simulink library "marine_gnc"  (Simulink 7.4)
settings: Solver=ode45  SolverMode=SingleTasking  StartTime=0.0  StopTime=10.0  RelTol=1e-3
undefined symbols (not defined in the file or in its folder): CN_data, CX_data, CY_data, D, G, K_supply, kt2ms, M, MA, magnitude, marine, Models, MRB, order, pathlength, RAO_Amp, RAO_Dir, RAO_Freq, RAO_Phase, RAO_Vel, RAO_yaw_back, RAO_yaw_quant, RAO_yaw_quantization_flag, rho_a, Semi, sub, T_supply, table, Tanker, vessel, Vessels
libraries: marine_gnc x64, simulink x39, cybersealib x1
(part 1 of 6)
settings Model: Creator=tristan  LastModifiedBy=Thor

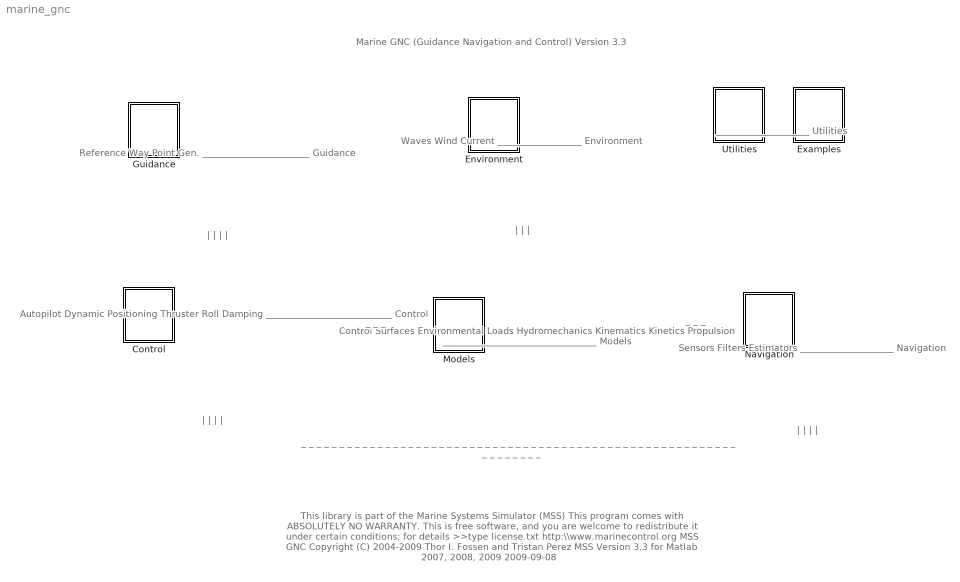
== system marine_gnc ==
  note: Marine GNC (Guidance Navigation and Control) Version 3.3
  note: Reference
      |                      Way Point Gen.
      |
      |
      | _______________________
      | Guidance
  note: Control Surfaces
      |                              Environmental Loads
      |                      Hydromechanics
      |           Kinematics
      |      Kinetics
      |            Propulsion
      | _________________________________
      | Models
  note: Autopilot
      |                          Dynamic Positioning
      |     Thruster
      |              Roll Damping
      | ___________________________
      | Control
  note: Waves
      |                    Wind
      |                        Current
      |
      | __________________
      | Environment
  note: |
      | |
      | |
  note: _ _ _
  note: _ _ _
  note: |
      | |
      | |
      | |
  note: |
      | |
      | |
      | |
  note: |
      | |
      | |
      | |
  note: _ _ _ _ _ _ _ _ _ _ _ _ _ _ _ _ _ _ _ _ _ _ _ _ _ _ _ _ _ _ _ _ _ _ _ _ _ _ _ _ _ _ _ _ _ _ _ _ _ _ _ _ _ _ _ _ _ _ _ _ _ _ _ _ _
  note: Sensors
      |                    Filters
      |                           Estimators
      |
      | ____________________
      | Navigation
  note: This library is part of the Marine Systems Simulator (MSS)
      | This program comes with ABSOLUTELY NO WARRANTY. This is free software,
      | and you are welcome to redistribute it under certain conditions; for details
      | >>type license.txt
      |
      |  http:\\www.marinecontrol.org
      |
      | MSS GNC  Copyright (C) 2004-2009 Thor I. Fossen and Tristan Perez
      |  MSS Version 3.3 for Matlab 2007, 2008, 2009
      | 2009-09-08
  note: ____________________
      | Utilities
  Control : Subsystem
  Environment : Subsystem
  Examples : Subsystem  AncestorBlock=Marine_GNC/Support and Examples
  Guidance : Subsystem
  Models : Subsystem
  Navigation : Subsystem
  Utilities : Subsystem

== system marine_gnc/Control ==
  Autopilots : Subsystem
  "Dynamic  Positioning " : Subsystem
  Thruster : Subsystem

== system marine_gnc/Environment ==
  Current : Subsystem
  Waves : Subsystem
  Wind : Subsystem

== system marine_gnc/Examples ==
  Applications : Subsystem
  Vessels : Subsystem

== system marine_gnc/Guidance ==
  Reference model : Subsystem  mask(3rd-order reference model){v_max=1.0, zeta_d=1.0, w_d=0.1}
      mask prompts: v_max "Max. velocity:"; zeta_d "Relative damping ratio:"; w_d "Natural frequency:"
      mask help: 3rd-order reference model with velocity saturation.
      mask Display:
      | disp('3rd order \nLP-filter')
      | port_label('output', 3, 'acc_d')
      | port_label('output', 2, 'vel_d')
      | port_label('output', 1, 'mag_d')
      | port_label('input', 1, 'ref')
  Way-point guidance block : Subsystem  mask(Guidance){x_vector=[-800 -500 -200 -50 -200 -250 200 500 500 300 0 -300 -600], y_vector=[100 1800 2000 1500 1000 100 1000 300 -250 -200 100 -600 -1000], method=5th order polynomial, drawmode=off, stop=on, mode=Acc, start=[100 0], final=[0 100], constraint=off}
      mask prompts: x_vector "X value"; y_vector "Y value"; method "Computation method for path generation"; drawmode "Draw an extra plot showing the path with waypoints"; stop "Stop simulation when last waypoint is reached"; mode "Use constraints on acceleration or velocity in the endpoints"; start "Constraints in first waypoint [x, y]. (Only applicable for cubic splines)"; final "Constraints in last waypoint [x, y]. (Only applicable for cubic splines)"; constraint "Use constraints on the derivatives (Only applicable for 5th order)"
      mask help:
      | Way-Point Guidance Block
      | Author:  Jorgen Corneliussen
      | Date:     20 November 2002
      |
      | Creates a three times differentiable path between the waypoints provided. The user can choose between cubic splines and polinomial interpolation.
      |
      | NOTE: You have to supply the actual waypoints for the path generation.
      mask init:
      | if method == 1
      | 	[table, pathlength] = order3(x_vector,y_vector, drawmode, mode, start(1), final(1), start(2), final(2));
      | elseif method == 2
      | 	[table, pathlength] = order5(drawmode, constraint, x_vector, y_vector);
      | else
      | 	disp('Error in block initialization')
      | end
      mask Help:
      | <p>Way-Point Guidance Block<br>
      |   Author: Jorgen Corneliussen<br>
      |   Date: 20 November 2002</p>
      | <ul>
      |   <li> The input vectors must be of the same length, and contain the coordinates
      |     of the waypoints.</li>
      |   <li>If chosen, the block can draw an extra plot showing the path and the waypoints.</li>
      |   <li> The field &quot;Computation method&quot; allows the user to choose between
      |     a third and fifth order polynomal for path generation. </li>
      |   <li>If &quot;Stop simulation&quot; is not checked, the velocity input to the
      |     block is set to zero when the last waypoint is reached. </li>
      |   <li>For the third order algorithm, the user can choose between having endpoint
      |     constraints in velocity or acceleration. The values must be provided in the
      |     specified fields.</li>
      |   <li>For the fifth order polynomial, the user can choose to constrain the derivatives
      |     in the waypoints. This might in some cases reduce oscillations.<br>
      |   </li>
      | </ul>
      mask StyleString: edit,edit,popup(Cubic spline|5th order polynomial),checkbox,checkbox,popup(Vel|Acc),edit,edit,checkbox
      mask Display:
      | image(imread('compass.jpg'))
      | 
      | color('black'); port_label('output', 1, 'xy')
      | color('black'); port_label('output', 2, 'eta_vec')
      | color('black'); port_label('output', 3, 'vs_tot')
      | 
      | color('black'); port_label('input', 1, 'ud_total')
      | color('black'); port_label('input', 2, 'theta')
  "Zig-Zag test rudder command " : Subsystem  mask(Z- Manoeuvre test or Zig-Zag test){RL=}
      mask prompts: RL "Maximum rudder angle [rad]:"
      mask help:
      | This block generates the rudder command for a Z-manoeuvre test
      | IMO A601, ITTC 1975, SNAME 1989.
      | Copyright (C) 2005 NTNU
      |  Author: Tristan Perez

== system marine_gnc/Models ==
  " Kinematics" : Subsystem
  " Kinetics " : Subsystem
  Control Surfaces : Subsystem
  Environmental Loads : Subsystem
  Hydromecanics : Subsystem
  Propulsion : Subsystem

== system marine_gnc/Navigation ==
  Filters : Subsystem
  Observers : Subsystem
  "Sensors " : Subsystem

== system marine_gnc/Utilities ==
  Dynamics : Subsystem
  Math Operations : Subsystem
  Simulation tools : Subsystem
  Visualization : Subsystem

== system marine_gnc/Control/Autopilots ==
  Heading autopilot : Subsystem  mask(Course Autopilot){T_nomoto=1, K_nomoto=1, Kp=1, Td=0, Ti=0}
      mask prompts: T_nomoto "Nomoto Time Constant: T"; K_nomoto "Nomoto gain: K"; Kp "Proportional Gain: Kp"; Td "Derivative Time: Td"; Ti "Integral Time: Ti"
      mask help: PID Autopilot with reference feedforward.
      mask Help: INPUTS: (1)  desired position, (2) desired velocity, (3) desired acceleration, (4) heading angle, (5) heading rate: OUTPUTS: (1) rudder angle
      mask Display: disp('PID\n tracking\n controller')

== system marine_gnc/Control/Dynamic  Positioning  ==
  DP controller : Subsystem  mask(Nonlinear DP Controller){Kp=diag([1 1 1]), Kd=diag([1 1 1]), Ki=diag([1 1 1])}
      mask prompts: Kp "Proportional Gain Matrix: Kp"; Kd "Derivative Gain Matrix: Kd"; Ki "Integral Gain Matrix: Ki"
      mask help: Nonlinear PID controller for Set-Point Reulation in Surge, Sway and Yaw
      mask Help:
      | The nonlinear  PID controller uses the rotation matrix in yaw for proper scaling of the surge, sway and yaw gains as a function of the yaw angle.
      | INPUTS: (1) eta_ref, (2) eta, (3) nu. OUPUTS: (1) tau.
      mask Display: disp('Nonlinear PID\n set-point controller')

== system marine_gnc/Control/Thruster ==

== system marine_gnc/Environment/Current ==
  North-East current : Subsystem

== system marine_gnc/Environment/Waves ==
  " Gaussian Random Process" : Subsystem  AncestorBlock=|  mask(Gaussian Random Process as a Sum of Sinusoids){areg=, freq=, phases=}
      | dcmv/Environmental
      | Disturbances/Fourier representation of 
      | a Gaussian Random Process
      mask prompts: areg "Vector of Amplitudes [A1;A2;...]:"; freq "Vector of frequencies [W1;W2;...]  [rad/sec]:"; phases "Vector of random phases [P1;P2;...]  [rad]:"
      mask help:
      | y = Sum_i  Ai *cos(w_i*t+ Phi_i)
      | Input:
      |  t --Simulation time from a clock block
      | Output:
      |  y--Realization of the random process y(t) (time series)
      | Dependency: None
      |
      | Copyright (C), NTNU  2004
      | Author: Tristan Perez
      mask Help: web(['file:///' which('Help_Gaussian_Random_Process.htm')]);
      mask Display:
      | plot([-ones(1,17)
      | 	0.6333
      |      -1.5315
      |    -0.5146
      |     0.5573
      |     1.2590
      |     1.8899
      |     1.5451
      |    -0.1055
      |    -1.0617
      |    -1.3645
      |    -1.3826
      |    -1.2742
      |     0.3850
      |     1.0225
      |     1.1108
      |     1.1270
      |     0.3762
      |    -0.6570
      |    -1.1216
      |    -0.2885
      |     0.9176
      |     0.7826
      |    -0.3229
      |    -1.2406
      |    -0.9331
      |    -0.2407
      |     0.4134
      |     0.8612
      |     0.3025
      |     0.2761
      |     0.3856
      |     0.3689
      |    -0.0188
      |     0.3654
      |    -0.4219
      |    -1.0260
      |    -1.3896
      |    -0.6530
      |     0.2512
      |     1.0351
      |     1.6496
      |     0.8313
      |    -1.2176
      |    -1.0937
      |     0.0268
      |     1.0361
      |     1.1728
      |    -0.2176
      |    -0.6390
      |    -1.1209
      |    -1.0516
      |    -0.4193
      |     0.7858
      |     0.8509
      |     0.4288
      |     0.0431
      |     0.0587 -ones(1,15
      | 	)])
      | port_label('input',1,'time')
      | port_label('output',1,'y')
  Encounter frequency correction : Subsystem
      mask Type: Encounter frequency correction
      mask Description:
      | This block transforms the frequencies and wave numbers in the Waves bus generated by the MSS Waves block to encounter frequencies and encounter wave numbers using the transformation:
      | 
      | Omega_e = Omega - U*Omega^2*cos(Psi_r)/g
      | 
      | where U is the vessel forward speed, Psi_r is the angle of the waves relative to the vessel.
      | 
      | Inputs:
      | Waves - Bus of harmonic wave components generated by the MSS Waves block.
      | U          - Forward speed of the reference frame relative to NED (m/s) (Usually the low-frequency speed of the vessel)
      | Psi       - Yaw orientation of the reference frame relative to NED (rad) (Usually the low-frequency heading of the vessel)
      | 
      | Outputs:
      | Waves - Bus of harmonic wave components with corrected wave frequencies and wave numbers.
      | 
      | Copyright (C) 2005, NTNU
      | Author: Øyvind Notland Smogeli
  Linear 2nd-order  wave spectrum : Subsystem  mask{sigma=1, w_0=1, lambda=0.1}
      mask prompts: sigma "Wave spectrum gain: sigma  (m)"; w_0 "Wave spectrum peak frequency: w_0  (rad/s)"; lambda "Rrelative damping ratio: lambda"
      mask init:
      | w = 0.01:0.1:3*w_0;
      mask Display:
      | plot(w,4*w_0*sigma^2.*w.^2./((w_0^2-w.^2).^2+4*(lambda*w_0.*w).^2))
      | port_label('input', 1, 'w')
      | port_label('output', 1, 'y')
  W_wave 2 W_enc (no absolute value) : Subsystem
      mask Type: Wave frequency to Encounter Frequency
      mask Description:
      | This block implements the transformation:
      | 
      | We = W -U W^2 cos(Enc Aang) /g
      | 
      | Inputs:
      | U---forward speed of the reference frame (m/sec) (sually the speed of the vessel)
      | W--vector of wave frequencies (rad/sec)
      | Enc. Angle-- (rad) convention: 0-following seas; pi/2-port beam seas; pi-head seas
      | 
      | Outputs:
      | We--vector of encounter frequencies (rad/sec).
      | Ke-- vector of encounter wave numbers (Ke = We^2/g deep water assumption)
      | Copyright (C) 2005, NTNU
      | Author: Tristan Perez
      mask Help:
      | <p>This block implements the transformation: <br>
      | <br>
      | We = W -U W^2 cos(Enc Ang) /g <br>
      | <br>
      | Inputs:<br>
      | U---forward speed of the reference frame (m/sec) (Usually the speed of the
      | vessel)<br>
      | W--vector of wave frequencies (rad/sec)<br>
      | Enc. Angle-- (rad) convention: 0-following seas; pi/2-port beam seas; pi-head
      | seas<br>
      | <br>
      | Outputs:<br>
      | We--vector of encounter frequencies (rad/sec).<br>
      | Ke-- vector of encounter wave numbers (Ke = We^2/g deep water assumption)<br>
      | Copyright (C) 2005, NTNU<br>
      | Author: Tristan Perez </p>
  Wave velocitycalc : Subsystem
      mask Type: Wave velocitycalc
      mask Description: Caclulates the wave-induced water velocity in NED coordinates and surface elevation Zeta at the point [x y z] in NED. The Waves bus generated by the Waves module is needed as input.
  Waves : Subsystem  mask(Waves){spectrum_type=ITTC, disp_flag=on, plot_spectrum=off, plot_realization=off, hs=0.8, omega_peak=0, psi_mean=0, gamma=-1, spread=2, depth=inf, nfreq=20, ndir=10, energylim=0.005, freq_cutoff=3, dir_cutoff=0, rand_seed=123, rand_freq=on, rand_dir=on, Zeta_a=0, Omega=0, Phase=0, Wavenum=0, Psi=0}
      mask prompts: spectrum_type "Spectrum type"; disp_flag "Display initialization info in workspace window"; plot_spectrum "Plot spectrum"; plot_realization "Plot sea state realization (time-consuming)"; hs "Significant wave height Hs (m)"; omega_peak "Peak frequency omega_0 (rad/s)"; psi_mean "Mean wave direction (rad)"; gamma "Spectrum peakedness factor [1,7], 3.3 default, 0 for using DNV value"; spread "Wave spreading factor (1,2,3,4,5)"; depth "Average water depth (m), use inf for deep water"; nfreq "Number of frequencies in grid (recommended > 20)"; ndir "Number of directions in grid, 1 for long-crested waves"; energylim "Wave component energy limit [0 1] or number of waves (e.g. 50)"; freq_cutoff "Frequency cutoff factor [1.5, 5], default 3"; dir_cutoff "Direction cutoff [0, 3pi/8], default 0"; rand_seed "Random seed"; rand_freq "Random frequencies"; rand_dir "Random directions"; Zeta_a "Amplitude vector 'Zeta_a' (m)"; Omega "Frequency vector 'Omega' (rad/s)"; Phase "Phase vector 'Phase' (rad)"; Wavenum "Wavenumber vector 'Wavenum' (1/m)"; Psi "Direction vector 'Psi'  (rad)"
      mask help:
      | Calculate harmonic wave component parameters from a wave spectrum.
      | - Input one wave direction in the mask to get long-crested waves.
      | - Input zero peak frequency to get an expectation value from north sea statistical data.
      | - Input an integer > 1 for energylim to set the number of wave components fixed to nwaves = energylim.
      |
      | Copyright (C) 2004 NTNU
      | Author: Oyvind Notland Smogeli
      mask init:
      | if spectrum_type < 4
      | 	[Zeta_a, Omega, Phase, Wavenum, Psi] = Wave_init(spectrum_type, hs, omega_peak, psi_mean,...
      | 	gamma, spread, depth, nfreq, ndir, energylim, freq_cutoff, dir_cutoff, rand_freq, rand_dir,...
      | 	rand_seed, plot_spectrum, plot_realization, disp_flag);
      | end
      mask Help:
      | <font face="Arial">
      | <b>Project:</b> Marine Systems Simulator: MSS<br>
      | <br>
      | Define harmonic wave components describing the sea state by extracting
      | components from a given frequency and direction spectrum. The output from the
      | block is a bus containing the following wave parameter vectors:</font></p>
      | <p><font face="Arial"><b>Zeta_a</b>: Vector of harmonic wave amplitudes [m]<br>
      | <b>Omega: </b>Vector of harmonic wave frequencies [rad/s]<br>
      | <b>Phase: </b>Vector of harmonic wave phases (random) [rad]<br>
      | <b>Wavenum:</b> Vector of harmonic wave numbers [1/m]<br>
      | <b>Psi: </b>Vector of harmonic wave directions [rad]</font></p>
      | <p><font face="Arial">The time series of sea surface elevation Zeta(x,y,t) can
      | be obtained as</font></p>
      | <p><font face="Arial">Zeta(x,y,t) = Sum( Zeta_a(i)*cos(Omega(i)*t + Phase(i) - Wavenum(i)*(x*cos(Psi(i))
      | + y*sin(Psi(i)))) )</font></p>
      | <p><font face="Arial">where the sum is taken from i = 1 to i = n and n is the number of harmonic
      | wave components.</font></p>
      | <p>&nbsp;</p>
      | <p><font face="Arial">Input one wave direction to get long-crested waves.<br>
      | <br>
      | If the peak frequency is set to zero, then the peak frequency is obtained from
      | the sugnificant wave height usign a formula for the North Sea (Norsok):</font></p>
      | <p><font face="Arial">w0 = 2*pi/(4.883 + 2.68*Hs^0.54);</font></p>
      | 
      | <p>&nbsp;</p>
      | <p><font face="Arial">The energy limit (energylim) should be defined either as a positive factor
      | between 0 and 1, or as a positive integer. In the first case it will
      | discard all wave components with energy content less than this ratio of the
      | total energy content of the sea state. A recommended value is 0.005 or lower. In
      | the second case it will keep the nwaves = energylim most significant waves.</font></p>
      | <p>&nbsp;</p>
      | <p><font face="Arial">The wave elevation Zeta(x,y,t) at time t and at the coordinate (x,y) is found from the output vectors as:</font></p>
      | <p>&nbsp;</p>
      | <p><font face="Arial" color="#800000">References</font><ul>
      |   <li><font face="Arial">Sørensen, A.J. (2005) Lecture notes of TMR4240 &quot;Marine Cybernetics - Modelling and Control&quot;</font>
      |   <font face="Arial">Dept of Marine Technology NTNU.</font></li>
      |   <li><font face="Arial">Johannessen, K., T. S. Meling, S. Haver. Joint
      |   Distribution for Wind and<br>
      |   Waves in the Northern North Sea. IJOPE Vol. 12, No. 1, March 2002</font></li>
      |   <li>&nbsp;</li>
      |   </ul>
      | <p><font face="Arial">Johannessen, K., T. S. Meling, S. Haver. Joint
      | Distribution for Wind and<br>
      | Waves in the Northern North Sea. IJOPE Vol. 12, No. 1, March 2002</font><p>&nbsp;<p>
      |   <font face="Arial"><b>Author:</b> Øyvind Smogeli, September 2004 </font>
      | <p>&nbsp;</p>
      | <p>&nbsp;</p>
      mask StyleString: popup(ITTC|Jonswap|Torsethaugen|Predefined waves),checkbox,checkbox,checkbox,edit,edit,edit,edit,edit,edit,edit,edit,edit,edit,edit,edit,checkbox,checkbox,edit,edit,edit,edit,edit
      mask CallbackString: Wave_callback;||||||||||||||||||||||

== system marine_gnc/Environment/Wind ==
  Wind : Subsystem  mask(Wind){page=1, Par_Wind_slowlyvar=off, Par_Wind_gust=off, Par_Wind_V=10, Par_Wind_angle=0, Par_Wind_spectrum_type=1, Par_Wind_z=10, Par_Wind_sample_time=0.1, Par_Wind_speed_T=10, Par_Wind_angle_T=10, Par_Wind_speed_noise_pow=1, Par_Wind_angle_noise_pow=0.01, Par_Wind_speed_rand_max=1, Par_Wind_angle_rand_max=pi/4, Par_Wind_speed_seed=123, Par_Wind_angle_seed=321, Par_Wind_phase_seed=1532, Par_Wind_kappa_H=0.0026, Par_Wind_L=1800, Par_Wind_minfreq=1E-4, Par_Wind_maxfreq=0.1, Par_Wind_nfreq=100}
      mask prompts: Par_Wind_slowlyvar "Include slowly-varing wind velocity and direction"; Par_Wind_gust "Include wind gust"; Par_Wind_V "Mean wind velocity [m/s]"; Par_Wind_angle "Mean wind angle [rad]"; Par_Wind_spectrum_type "Wind gust spectrum type"; Par_Wind_z "Height over water surface [m (for NORSOK wind spectrum)]"; Par_Wind_sample_time "Wind sample time [s]"; Par_Wind_speed_T "Wind speed time constant [s]"; Par_Wind_angle_T "Wind angle time constant [s]"; Par_Wind_speed_noise_pow "Wind speed noise power"; Par_Wind_angle_noise_pow "Wind angle noise power"; Par_Wind_speed_rand_max "Wind speed saturation [m/s] (max random variation about mean)"; Par_Wind_angle_rand_max "Wind angle saturation [rad] (max random variation about mean)"; Par_Wind_speed_seed "Wind speed random seed"; Par_Wind_angle_seed "Wind angle random seed"; Par_Wind_phase_seed "Wind gust phase seed"; Par_Wind_kappa_H "Sea surface drag coefficient for Harris wind spectrum (0.0026)"; Par_Wind_L "Scaling length for Harris wind spectrum (1800)"; Par_Wind_minfreq "Minimum frequency in gust [Hz] (1E-4)"; Par_Wind_maxfreq "Maximum frequency in gust [Hz] (0.1)"; Par_Wind_nfreq "Number of frequency components"
      mask help:
      | Generates wind speed and direction based on the mean angle and mean wind speed at 10 meters height. The total velocity is composed of a slowly-varying mean superposed with gusts based on a chosen wind spectrum. The direction is slowly-varying based on a random process.
      |
      | The wind spectrum types are:
      |
      | 1) Harris         (based on measurements over land)
      | 2) NORSOK   (based on measurements from the North Sea)
      mask Help:
      | <b>Part of the Marine Systems Simulator: MSS</b><p>Generate wind speed and direction based on the mean angle and mean wind
      | speed at 10 meters height. The total velocity is composed of a slowly-varying
      | mean superposed with gusts based on a chosen wind spectrum. The direction is
      | slowly-varying based on a random process.<br>
      | <br>
      | The wind spectrum types are:<br>
      | <br>
      | 1) Harris (based on measurements over land)<br>
      | 2) NORSOK (based on measurements from the North Sea)</p>
      | <p>The wind gust from the Harris spectrum is uniform over the height, whereas
      | the wind gust from the NORSOK spectrum varies with the height.</p>
      | <p>The random variation of the mean speed and angle can be limited by two saturation
      | parameters, which define the maximum random deviation from the mean value.<p><b>Outputs:
      | </b> </p>
      | <p>angle: [rad] Wind angle in the n-frame<br>
      | speed: [m/s] Wind velocity in the n-frame<p>
      | <b>Copyright NTNU 2005</b></p>
      | <p><b>Author:</b> Oyvind N. Smogeli, 2005-05-03</p>
      mask StyleString: popup(1|2),checkbox,checkbox,edit,edit,popup(1|2),edit,edit,edit,edit,edit,edit,edit,edit,edit,edit,edit,edit,edit,edit,edit,edit
      mask CallbackString: MSS_mask_page(12);|||||||||||||||||||||

== system marine_gnc/Examples/Applications ==
  Autopilot - Kalman filter based wave filter using only compass : Subsystem  AncestorBlock=marine/Examples/Autopilot - Kalman filter based wave filter using only compass  mask{A=}
      mask prompts: A "Needed to invoke OpenFcn from the browser:"
      settings: OpenFcn=sfundemo_open('demowf3')
      mask Display: disp('Autopilot - \n Kalman filter based\n wave filter using\n only compass');
  Autopilot - passive wave filter using compass/gyro : Subsystem  mask{A=}
      mask prompts: A "Needed to invoke OpenFcn from the browser:"
      settings: OpenFcn=sfundemo_open('demowf2')
      mask Display:
      | disp('Autopilot - \n passive wave filter\n
      | using compass/gyro');
  Autopilot - passive wave filter using only compass : Subsystem  mask{A=}
      mask prompts: A "Needed to invoke OpenFcn from the browser:"
      settings: OpenFcn=sfundemo_open('demowf1')
      mask Display:
      | disp('Autopilot - \n passive wave filter \n
      | using only compass');
  DP system for CyberShipII : Subsystem  mask{A=}
      mask prompts: A "Needed to invoke OpenFcn from the browser:"
      settings: OpenFcn=sfundemo_open('demoCS2')
      mask Display: disp('DP system for \n CyberShipII');
  DP system for semi-submersible : Subsystem  mask{A=}
      mask prompts: A "Needed to invoke OpenFcn from the browser:"
      settings: OpenFcn=sfundemo_open('demorig')
      mask Display: disp('DP system for\n semi-submersible');
  Simulink interface for m-file vessel models : Subsystem  mask{A=}
      mask prompts: A "Needed to invoke OpenFcn from the browser:"
      settings: OpenFcn=sfundemo_open('demomf')
      mask Display:
      | disp('Simulink interface for\n
      | m-file vessel models');
  Thruster configuration demo for a supply vessel : Subsystem  mask{A=}
      mask prompts: A "Needed to invoke OpenFcn from the browser:"
      settings: OpenFcn=sfundemo_open('demothr')
      mask Display: disp('Thruster configuration\n for a supply vessel');
  Waves : Subsystem  mask{A=}
      mask prompts: A "Needed to invoke OpenFcn from the browser:"
      settings: OpenFcn=sfundemo_open('demo_waves')
      mask Display: disp('Waves');
  Way-point guidance system : Subsystem  mask{A=}
      mask prompts: A "Needed to invoke OpenFcn from the browser:"
      settings: OpenFcn=sfundemo_open('demowpt')
      mask Display: disp('Way-point guidance\n system');
  Zig-zag Test : Subsystem  AncestorBlock=marine_gnc/Examples/Applications/Autopilot - passive wave filter using only compass  mask{A=}
      mask prompts: A "Needed to invoke OpenFcn from the browser:"
      settings: OpenFcn=sfundemo_open('demo_nv_mano')
      mask Display: disp('Naval Vessel  \n Manoeuvring');

== system marine_gnc/Examples/Vessels ==
  note: Interface to m-file models
  note: Low-Speed Models (6 DOF) 6 DOF interface for 3 DOF models
  note: Low-Speed Models (3 DOF)
  6 DOF supply vessel interface : Subsystem  AncestorBlock=marine/Models/Vessels/6 DOF supply vessel interface
      mask Display: disp('6 DOF interface\n to 3 DOF vessel\n models')
  CyberShipII : Subsystem  AncestorBlock=marine/Models/Vessels/CyberShipII  LoadFcn=initCS2
      mask Display:
      | image(imread('figs/cs.jpg'))
      | color('white'); port_label('output', 1, 'eta')
      | color('white');port_label('output', 2, 'nu')
      | color('white'); port_label('input', 1, 'tau')
  Mariner class cargo ship  (2nd -order) : Subsystem  AncestorBlock=|  mask(Container ship (2nd-order model)){rate_max=5*(pi/180), delta_max=20*(pi/180), K=0.185, T1=118, T2=7.8, T3=18.5}
      | marine/Models/Vessels/Mariner class cargo ship
      |  (2nd -order)
      mask prompts: rate_max "Max rudder rate: rate_max (rad/s)"; delta_max "Max rudder angle: delta_max (rad)"; K "Gain constant: K (1/s)"; T1 "Time constant: T1 (s)"; T2 "Time constant: T2 (s)"; T3 "Time constant: T3 (s)"
      mask Display:
      | image(imread('figs/container.jpg'))
      | color('white'); port_label('output', 1, 'psi')
      | color('white'); port_label('output', 2, 'r')
      | color('white'); port_label('output', 3, 'delta')
      | color('white'); port_label('input', 1, 'delta_c')
  Naval Vessel 4DOF (360ton) : Subsystem  mask(Naval Vessel Nonlinear Manoeuvring Model){ic=[kt2ms(15),0,0,0,0,0]'}
      mask prompts: ic "Initial Condition x=[u,v,p,r,phi,psi]"
      mask help:
      | Naval Vessel Model in 4DOF (surge,sway, roll, and yaw)
      | Input:
      | Tau -- vector of forces [X,Y,K,N]' in Newtons
      |
      | Output:
      | Eta --  [phi,psi]'  Euler angles [rad]
      | Nu  --  [u,v,p,r]   Linear and angular velocities in the body-fixed frame.
      |
      | Copyright 2005 NTNU
      | Author: Tristan Perez
      mask Help:
      | <p><font face="Arial">This is nonlinear manoeuvring model un 4DOF. This model
      | has been implemented usign the GNC vessel model block, and the </font>
      | <font face="Courier">m</font><font face="Arial"> file associated with the model
      | is </font></p>
      | <p><font face="Courier">mss\vessel_models\nv_nl_model.m</font></p>
      | <p><font face="Arial">All the hydrodynamic data is in the above file.&nbsp; For
      | an example of use see&nbsp; the following demo:</font></p>
      | <p><font face="Courier">mss\simulink\demos\demo_nv_mano.mdl</font></p>
      mask Display:
      | image(imread('nvessel.jpg'))
      | color('white'); port_label('output', 1, 'Eta')
      | color('white');port_label('output', 2, 'Nu')
      | color('white'); port_label('input', 1, 'Tau')
  Semi-sub : Subsystem  AncestorBlock=marine/Models/Vessels/Semi-sub  InitFcn=load MDGmodels/rig  mask(Semi-submersiblel (6 DOF)){D=D, G=G, MA=MA, MRB=MRB}
      mask prompts: D "Linear damping matrix: D"; G "Spring matrix G:"; MA "System inertia added mass matrix: M"; MRB "System inertia rigid-body matrix"
      mask help:
      | Semi-submersible low-speed model for DP.
      |
      | Inputs:
      |
      |    tau = 6 DOF control input vector (generalized force)
      |
      | Outputs:
      |
      |    eta = [x, y, z, phi, theta, psi]'
      |    nu  = [u, v, w, p, q, r]'
      mask Display:
      | image(imread('figs/semisub.jpg'))
      | color('black'); port_label('output', 1, 'eta')
      | color('black'); port_label('output', 2, 'nu')
      | color('black'); port_label('input', 1, 'tau')
      | color('black'); port_label('input', 2, 'nu_c')
  Supply vessel : Subsystem  AncestorBlock=marine/Models/Vessels/Supply vessel  mask(Supply Vessel (surge, sway and yaw)){D=[5.0242e4 0 0; 0 2.7229e5 -4.3933e6; 0 -4.3933e6 4.1894e8], Minv=inv( [5.3122e6 0 0; 0 8.2831e6 0; 0 0 3.7454e9] )}
      mask prompts: D "Linear damping matrix: D"; Minv "Inverse inertia matrix: Minv"
      mask help:
      | DP model
      |
      | Inputs:
      |
      |    tau = 3 DOF control input vector (generalized force)
      |
      | Outputs:
      |
      |    eta = [x, y, psi]'
      |    nu  = [u, v, r]'
      mask Display:
      | image(imread('figs/supply.jpg'))
      | color('black'); port_label('output', 1, 'eta')
      | color('black'); port_label('output', 2, 'nu')
      | color('black'); port_label('input', 1, 'tau')
  Tanker (1st-order) : Subsystem  mask(Tanker (Nomoto 1st.-order)){rate_max=5*(pi/180), delta_max=20*(pi/180), K=-0.019, T=-153.7}
      mask prompts: rate_max "Max rudder rate: rate_max (rad/s):"; delta_max "Max rudder angle: delta_max  (rad)"; K "Gain constant: K (1/s)"; T "Time constant: T (s)"
      mask help:
      | Tanker: Nomoto 1st-order model
      |
      | Input:
      |
      |   delta_c = rudder angle command (rad)
      |
      | Outputs:
      |
      |    psi    = yaw angle (rad)
      |    r        = yaw rate (rad)
      |    delta = rudder angle from steering machine (rad)
      mask Display:
      | image(imread('figs/tanker.jpg'))
      | color('white'); port_label('output', 1, 'psi')
      | color('white'); port_label('output', 2, 'r')
      | color('white'); port_label('output', 3, 'delta')
      | color('white'); port_label('input', 1, 'delta_c')
  Tanker (2nd-order) : Subsystem  AncestorBlock=marine/Models/Vessels/Tanker (2nd-order)  mask(Tanker (Nomoto 2nd-order model)){rate_max=5*(pi/180), delta_max=20*(pi/180), K=-0.019, T1=-124.1, T2=16.4, T3=46}
      mask prompts: rate_max "Max rudder rate: rate_max (rad/s)"; delta_max "Max rudder angle: delta_max (rad)"; K "Gain constant: K (1/s)"; T1 "Time constant: T1 (s)"; T2 "Time constant: T2 (s)"; T3 "Time constant: T3 (s)"
      mask help:
      | Tanker: Nomoto 2nd-order model
      |
      | Input:
      |
      |   delta_c = rudder angle command (rad)
      |
      | Outputs:
      |
      |    psi    = yaw angle (rad)
      |    r        = yaw rate (rad)
      |    delta = rudder angle from steering machine (rad)
      mask Display:
      | image(imread('figs/tanker.jpg'))
      | color('white'); port_label('output', 1, 'psi')
      | color('white'); port_label('output', 2, 'r')
      | color('white'); port_label('output', 3, 'delta')
      | color('white'); port_label('input', 1, 'delta_c')
  m-file examples : Subsystem  AncestorBlock=marine/Models/Vessels/m-file examples
      mask Type: propeller
  m-file interface : Subsystem  mask(m-file vessel model interface){vessmodel=, dimx_model=}
      mask prompts: vessmodel "m-file vessel model"; dimx_model "dim x"
      mask help:
      | Inputs/outputs:
      |
      |    u   = control input vector
      |    xo = initial state vector
      |    x   = state vector of dimension dimx
      |
      | See help for details
      |
      | Copyright NTNU 2005
      | Author: T.I. Fossen
      | Modified: by T. Perez 2005-05-04
      mask Help:
      | <p><font face="Arial">Simulink interface to the GNC toolbox m-file vessel models.
      | The model of the vessel is specified in a matlab finction that takes a vector of
      | inputs (these could be forces, rudder angle, thruster demand, etc), and returns
      | the derivative of the state. </font></p>
      | <p><font face="Arial">In the mask just enter the name of the m-file without ' ',
      | and without the extension .m</font></p>
      | <p><font face="Arial">For example, <br>
      | </font><font face="Courier New"><font color="#0000FF">function</font> [Xdot] =
      | nv_nlin_model(in)<br>
      | <font color="#008000">%Noninear Model for describing surge, sway, roll and yaw
      | Interactions <br>
      | %of a multipurpose naval vessel. The surge is only coupled through a<br>
      | %centripetal terms.<br>
      | %<br>
      | %Use:[out]=nv_nlin_model(in)<br>
      | %<br>
      | %Output:<br>
      | % out= M^-1 [X,Y,K,N,p,r]' <br>
      | %<br>
      | %where<br>
      | % M is the total mass matrix<br>
      | % X is the surge force (hydrodynamic+centriperal+external)<br>
      | % Y is the sway force (hydrodynamic+centriperal+external)<br>
      | % K is the sway force (hydrodynamic+centriperal+external)<br>
      | % N is the sway force (hydrodynamic+centriperal+external)<br>
      | % p is the roll rate<br>
      | % r is the yaw rate<br>
      | % <br>
      | %Inputs:<br>
      | % in=[u,v p r phi psi,Xe,Ye,Ke,Ne]' <br>
      | %<br>
      | %where<br>
      | % u = surge velocity (m/s)<br>
      | % v = sway velocity (m/s)<br>
      | % p = roll velocity (rad/s)<br>
      | % r = yaw velocity (rad/s)<br>
      | % phi = roll angle (rad)<br>
      | % psi = yaw angle (rad)<br>
      | %<br>
      | % U = surge speed of the vessel [m/sec].<br>
      | % Xe is the surge external force (eg rudder and fin force)<br>
      | % Ye is the sway external force <br>
      | % Ke is the sway external force <br>
      | % Ne is the sway external force</font><br>
      | ...<br>
      | Xdot=...</font></p>
      | <p><font face="Arial">The above function corresponds to the demo of the naval
      | vessel performing manoeuvres (</font><font face="Courier New">demo_nv_mano.mdl</font><font face="Arial">).
      | For another example see the demo </font><font face="Courier New">demomf.mdl</font></p>
      mask Display: disp('GNC toolbox\n vessel model')

== system marine_gnc/Guidance/Reference model ==
  desired position : Inport  OutDataType=sfix(16)  OutScaling=2^0
  "    " : TransferFcn  Denominator=[1 0]
  "       " : Saturate  UpperLimit=v_max  LowerLimit=-v_max
  "         " : TransferFcn  Denominator=[1 0]
  Sum2 : Sum  Inputs=|+-  OutDataType=sfix(16)  OutScaling=2^0  SaturateOnIntegerOverflow=on  InputSameDT=on  OutDataTypeStr=Inherit: Same as first input
  Sum5 : Sum  Inputs=|+-  OutDataType=sfix(16)  OutScaling=2^0  SaturateOnIntegerOverflow=on  InputSameDT=on  OutDataTypeStr=Inherit: Same as first input
  damping : Gain  Gain=2*zeta_d*w_d  ParameterDataType=sfix(16)  ParameterScaling=2^0  OutDataType=sfix(16)  OutScaling=2^0  SaturateOnIntegerOverflow=on  OutDataTypeStr=Inherit: Same as input  ParamDataTypeStr=Inherit: Same as input
  low-pass filter : TransferFcn  Numerator=[w_d^3]  Denominator=[1 w_d]
  spring : Gain  Gain=w_d*w_d  ParameterDataType=sfix(16)  ParameterScaling=2^0  OutDataType=sfix(16)  OutScaling=2^0  SaturateOnIntegerOverflow=on  OutDataTypeStr=Inherit: Same as input  ParamDataTypeStr=Inherit: Same as input
  "desired position " : Outport  OutDataType=sfix(16)  OutScaling=2^0  InitialOutput=0
  desired velocity : Outport  Port=2  OutDataType=sfix(16)  OutScaling=2^0  InitialOutput=0
  desired acceleration : Outport  Port=3  OutDataType=sfix(16)  OutScaling=2^0  InitialOutput=0
  wires:
  damping/1 -> Sum5/2
  "         "/1 -> "       "/1
  "    "/1 -> "desired position "/1, spring/1
  spring/1 -> Sum2/2
  Sum2/1 -> Sum5/1
  low-pass filter/1 -> Sum2/1
  desired position/1 -> low-pass filter/1
  Sum5/1 -> "         "/1, desired acceleration/1
  "       "/1 -> damping/1, "    "/1, desired velocity/1

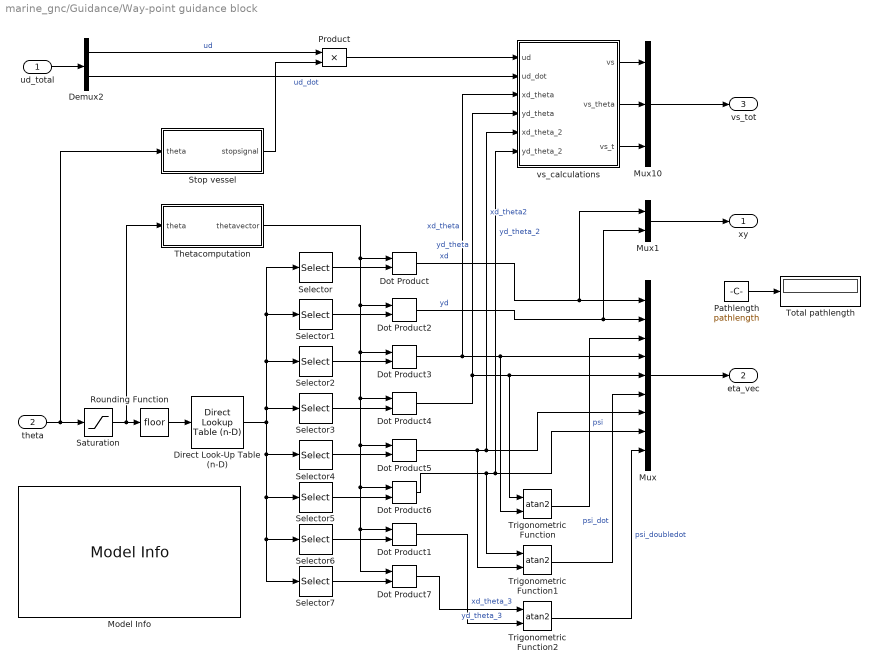
== system marine_gnc/Guidance/Way-point guidance block ==
  ud_total : Inport  PortDimensions=2  OutDataType=sfix(16)  OutScaling=2^0
  theta : Inport  Port=2  OutDataType=sfix(16)  OutScaling=2^0
  Demux2 : Demux  Outputs=2
  Direct Look-Up Table (n-D) : simulink/Lookup Tables/Direct Lookup Table (n-D)  maskTabDims=2  explicitNumDims=1  outDims=Column  tabIsInput=off  mxTable=table  clipFlag=None
  Dot Product{,1..7} (8 alike) : simulink/Math Operations/Dot Product  InputSameDT=on  OutDataType=sfix(16)  OutScaling=2^-10  DoSatur=off
  Model Info : simulink/Model-Wide Utilities/Model Info  InitialBlockCM=None  BlockCM=None  Frame=on  DisplayStringWithTags=|  HorizontalTextAlignment=Center  LeftAlignmentValue=0.5  SourceBlockDiagram=marine_gnc  TagMaxNumber=20
      | Guidance block.
      | Creates a three times differentiable path 
      | between the provided waypoints. The user 
      | can choose between cubic splines and a 
      | 5th order polynomial.
      | Author: Jorgen Corneliussen
      | Modified: %<ModifiedDate>
      | Version: %<ModelVersion>
  Mux : Mux  Inputs=9
  Mux1 : Mux  Inputs=2
  Mux10 : Mux  Inputs=3
  Pathlength : Constant  Value=pathlength  OutDataType=sfix(16)  OutScaling=2^0
  Product : Product  OutDataType=sfix(16)  OutScaling=2^0  SaturateOnIntegerOverflow=on  OutDataTypeStr=Inherit: Same as first input
  Rounding Function : Rounding
  Saturation : Saturate  UpperLimit=size(table,2) -0.001  LowerLimit=0
  Selector : Selector  InputPortWidth=size(table,1)  IndexOptions=Index vector (dialog)  Indices=[0*(size(table,1)/8)+1 :1*(size(table,1)/8)]  OutputSizes=1
  Selector1 : Selector  InputPortWidth=size(table,1)  IndexOptions=Index vector (dialog)  Indices=[1*(size(table,1)/8)+1 :2*(size(table,1)/8)]  OutputSizes=1
  Selector2 : Selector  InputPortWidth=size(table,1)  IndexOptions=Index vector (dialog)  Indices=[2*(size(table,1)/8)+1 :3*(size(table,1)/8)]  OutputSizes=1
  Selector3 : Selector  InputPortWidth=size(table,1)  IndexOptions=Index vector (dialog)  Indices=[3*(size(table,1)/8)+1 :4*(size(table,1)/8)]  OutputSizes=1
  Selector4 : Selector  InputPortWidth=size(table,1)  IndexOptions=Index vector (dialog)  Indices=[4*(size(table,1)/8)+1 :5*(size(table,1)/8)]  OutputSizes=1
  Selector5 : Selector  InputPortWidth=size(table,1)  IndexOptions=Index vector (dialog)  Indices=[5*(size(table,1)/8)+1 :6*(size(table,1)/8)]  OutputSizes=1
  Selector6 : Selector  InputPortWidth=size(table,1)  IndexOptions=Index vector (dialog)  Indices=[6*(size(table,1)/8)+1 :7*(size(table,1)/8)]  OutputSizes=1
  Selector7 : Selector  InputPortWidth=size(table,1)  IndexOptions=Index vector (dialog)  Indices=[7*(size(table,1)/8)+1 :8*(size(table,1)/8)]  OutputSizes=1
  Stop vessel : Subsystem
  Thetacomputation : Subsystem
  Total pathlength : Display
  Trigonometric Function : Trigonometry  Operator=atan2
  Trigonometric Function1 : Trigonometry  Operator=atan2
  Trigonometric Function2 : Trigonometry  Operator=atan2
  vs_calculations : Subsystem
  xy : Outport  OutDataType=sfix(16)  OutScaling=2^0
  eta_vec : Outport  Port=2  OutDataType=sfix(16)  OutScaling=2^0
  vs_tot : Outport  Port=3  OutDataType=sfix(16)  OutScaling=2^0
  wires:
  theta/1 -> Saturation/1, Stop vessel/1(theta)
  ud_total/1 -> Demux2/1
  Thetacomputation/1(thetavector) -> Dot Product/1, Dot Product2/1, Dot Product4/1, Dot Product5/1, Dot Product6/1, Dot Product7/1, Dot Product1/1, Dot Product3/1
  Dot Product/1 -> Mux/1, Mux1/1  "xd"
  Dot Product2/1 -> Mux/2, Mux1/2  "yd"
  Mux/1 -> eta_vec/1
  Dot Product3/1 -> Trigonometric Function/2, Mux/4, vs_calculations/3(xd_theta)  "xd_theta"
  Dot Product4/1 -> Mux/5, Trigonometric Function/1, vs_calculations/4(yd_theta)  "yd_theta"
  Dot Product5/1 -> Trigonometric Function1/2, Mux/7, vs_calculations/5(xd_theta_2)  "xd_theta2"
  Dot Product6/1 -> Trigonometric Function1/1, Mux/8, vs_calculations/6(yd_theta_2)  "yd_theta_2"
  Dot Product1/1 -> Trigonometric Function2/2  "xd_theta_3"
  Dot Product7/1 -> Trigonometric Function2/1  "yd_theta_3"
  Trigonometric Function/1 -> Mux/3  "psi"
  Trigonometric Function1/1 -> Mux/6  "psi_dot"
  Trigonometric Function2/1 -> Mux/9  "psi_doubledot"
  Mux10/1 -> vs_tot/1
  vs_calculations/1(vs) -> Mux10/1
  vs_calculations/3(vs_t) -> Mux10/3
  vs_calculations/2(vs_theta) -> Mux10/2
  Saturation/1 -> Rounding Function/1, Thetacomputation/1(theta)
  Selector/1 -> Dot Product/2
  Selector1/1 -> Dot Product2/2
  Selector2/1 -> Dot Product3/2
  Selector3/1 -> Dot Product4/2
  Selector4/1 -> Dot Product5/2
  Selector5/1 -> Dot Product6/2
  Selector6/1 -> Dot Product1/2
  Selector7/1 -> Dot Product7/2
  Direct Look-Up Table (n-D)/1 -> Selector/1, Selector1/1, Selector2/1, Selector3/1, Selector4/1, Selector5/1, Selector7/1, Selector6/1
  Rounding Function/1 -> Direct Look-Up Table (n-D)/1
  Demux2/1 -> Product/1  "ud"
  Product/1 -> vs_calculations/1(ud)
  Stop vessel/1(stopsignal) -> Product/2
  Demux2/2 -> vs_calculations/2(ud_dot)  "ud_dot"
  Mux1/1 -> xy/1
  Pathlength/1 -> Total pathlength/1

== system marine_gnc/Guidance/Zig-Zag test rudder command  ==
  Rudder Ang : Inport  OutDataType=sfix(16)  OutScaling=2^0
  "Yaw Ang  " : Inport  Port=2  OutDataType=sfix(16)  OutScaling=2^0
  Matrix Gain4 : Gain  Gain=[-1]  Multiplication=Matrix(K*u)  ParameterDataType=sfix(16)  ParameterScaling=2^0  OutDataType=sfix(16)  OutScaling=2^0  SaturateOnIntegerOverflow=on  OutDataTypeStr=Inherit: Same as input  ParamDataTypeStr=Inherit: Same as input
  Sum3 : Sum  OutDataType=sfix(16)  OutScaling=2^0  SaturateOnIntegerOverflow=on  InputSameDT=on  OutDataTypeStr=Inherit: Same as first input
  Switch : Switch  SaturateOnIntegerOverflow=on  InputSameDT=on
  test signal4 : Step  Time=0  After=RL  SampleTime=0
  "Rudder Command " : Outport  OutDataType=sfix(16)  OutScaling=2^0
  wires:
  test signal4/1 -> Switch/1, Matrix Gain4/1
  Matrix Gain4/1 -> Switch/3
  Sum3/1 -> Switch/2
  Rudder Ang/1 -> Sum3/1
  "Yaw Ang  "/1 -> Sum3/2
  Switch/1 -> "Rudder Command "/1

== system marine_gnc/Models/ Kinematics ==
  note: 3 DOF kinematic transformations
  note: 6 DOF kinematic transformations
  note: Euler angles
  6 DOF transformation : Subsystem
  Euler angles to inverse rotation matrix : Subsystem
      mask Type: Rbn
      mask Description:
      | Calculate the rotation matrix from NED coordinates to Body coordinates.
      | 
      | Input: Theta = [phi, theta, psi]'
      | 
      | Output: inv(Rzyx) (3x3)
      mask Help:
      | Calculate the rotation matrix from NED coordinates to Body coordinates.
      | 
      | Input: Theta = [phi, theta, psi]'
      | 
      | Output: inv(Rzyx) (3x3)
  Euler angles to rotation matrix : Subsystem
      mask Type: Euler2R
      mask Description: Determine the 3-by-3 rotation matrix from the Euler angles (roll, pitch, yaw) using the zyx convention.
      mask Display:
      | port_label('input',1,'theta')
      | port_label('output',1,'R')
  Euler angles to attitude transformation matrix : Subsystem
      mask Type: Euler2T
      mask Description: Determine the 3-by-3 attitude transformation matrix  from the Euler angles (roll, pitch, yaw).
      mask Display:
      | port_label('input',1,'theta')
      | port_label('output',1,'T')
  "Rotation matrix in yaw " : Subsystem
      mask Description:
      | b = R(psi)* a
      | 
      | where
      | 
      | input 1:    psi
      | input 2:    a - vector dim 3
      | output 1:  b - vector dim 3
      mask Display:
      | port_label('output', 1, 'R(psi)*v')
      | port_label('input', 1, 'psi')
      | port_label('input', 2, 'v')
  Transformation of generalized force : Subsystem
      mask Type: Transformation of generalized force
      mask Description:
      | Transforms a generalized force vector from one coordinate to a
      | new coordinate.
      | 
      | Takes the force vector in one point and the vector to the new point
      | as input, and gives the force vector in the new point as output.
      | 
      | Uses a Simulink version of the Hmtrx (inversed and transposed) gnc
      | matlab function.
  Transformation of generalized velocity : Subsystem
      mask Type: Velocity transformation
      mask Description:
      | Transforms a generalized velocity vector from one coordinate to a
      | new coordinate.
      | 
      | Takes the velocity vector in one point and the vector to the new point
      | as input, and gives the velocity vector in the new point as output.
      | 
      | Uses a Simulink version of the Hmtrx gnc matlab function.
      mask Help:
      | Transforms a generalized velocity vector from one coordinate to a
      | new coordinate.
      | 
      | Takes the velocity vector in one point and the vector to the new point
      | as input, and gives the velocity vector in the new point as output.
      | 
      | Uses a Simulink version of the Hmtrx gnc matlab function.
  Transposed rotation  matrix in yaw : Subsystem
      mask Description:
      | b = R'(psi)* a
      | 
      | where
      | 
      | input 1:    psi
      | input 2:    a - vector dim 3
      | output 1:  b - vector dim 3
      mask Display:
      | port_label('output', 1, 'R''(psi)*v')
      | port_label('input', 1, 'psi')
      | port_label('input', 2, 'v')

== system marine_gnc/Models/ Kinetics  ==
  3 DOF Eqs. of motion : Subsystem  mask(Equations of motion){CoriolisOnOff=on, nu0=[0 0 0], eta0=[0 0 0]}
      mask prompts: CoriolisOnOff "Coriolis and centripetal forces (check box to turn on)"; nu0 "Initial velocities (u,v,r)"; eta0 "Initial position/attitude (x,y,psi)"
      mask help:
      | 3 DOF equations of motion (surge, sway, roll and pitch)
      |
      |    eta_dot = J(eta)*nu
      |    (M_RB+M_A)*nu_dot + C_RB(nu)nu+C_A(nu_r)nu_r  =  tau
      |
      |    nu_r = nu-nu_c    (relative velocity)
      |    nu_c = [u_c, v_c, 0]  slowly-varying current velocity
      |
      | where nu = [u,v,r]' and eta = [x,y,psi]'
      |
      | The Coriolis and centripetal matrix C(nu) is computed automatically using the system inertia matrix M and nu,  see Chapter 3 in Fossen (2002) for details.
      |
      | T. I. Fossen (2002). Marine Control Systems: Guidance, Navigation and Control of Ships, Rigs and Underwater Vehicles, Marine Cybernetics AS, ISBN 82-92356-00-2
  6 DOF Eqs. of motion : Subsystem  mask(Equations of motion){CoriolisOnOff=on, nu0=[0 0 0 0 0 0], eta0=[0 0 0 0 0 0]}
      mask prompts: CoriolisOnOff "Coriolis and centripetal forces (check box to turn on)"; nu0 "Initial velocities (u,v,w,p,q,r)"; eta0 "Initial position/attitude (x,y,z,phi,theta,psi)"
      mask help:
      | 6 DOF equations of motion (surge, sway, heave, roll, pitch and yaw)
      |
      |    eta_dot = J(eta)*nu
      |    (M_RB+M_A)*nu_dot + C_RB(nu)nu+C_A(nu_r)nu_r  =  tau
      |
      |    nu_r = nu-nu_c    (relative velocity)
      |    nu_c = [u_c,v_c,w_c,0,0,0]  slowly-varying current velocity
      |
      | where nu = [u,v,w,p,q,r]'  and eta = [x,y,x,phi,theta,psi]'
      |
      | The Coriolis and centripetal matrix C(nu) is computed automatically using the system inertia matrix M and nu,  see Chapter 3 in Fossen (2002) for details.
      |
      | T. I. Fossen (2002). Marine Control Systems: Guidance, Navigation and Control of Ships, Rigs and Underwater Vehicles, Marine Cybernetics AS, ISBN 82-92356-00-2
  Support : Subsystem
